simulink model "ModeInt"  (R2018b)
settings: Solver=FixedStepDiscrete  StartTime=0.0  StopTime=10.0  FixedStep=0.01  RelTol=1e-3
undefined symbols (not defined in the file or in its folder): c, CmprtMdHMIReqTp1, e, IfVeSMSeStNumConfig, MdReqTp1
(part 2 of 4)

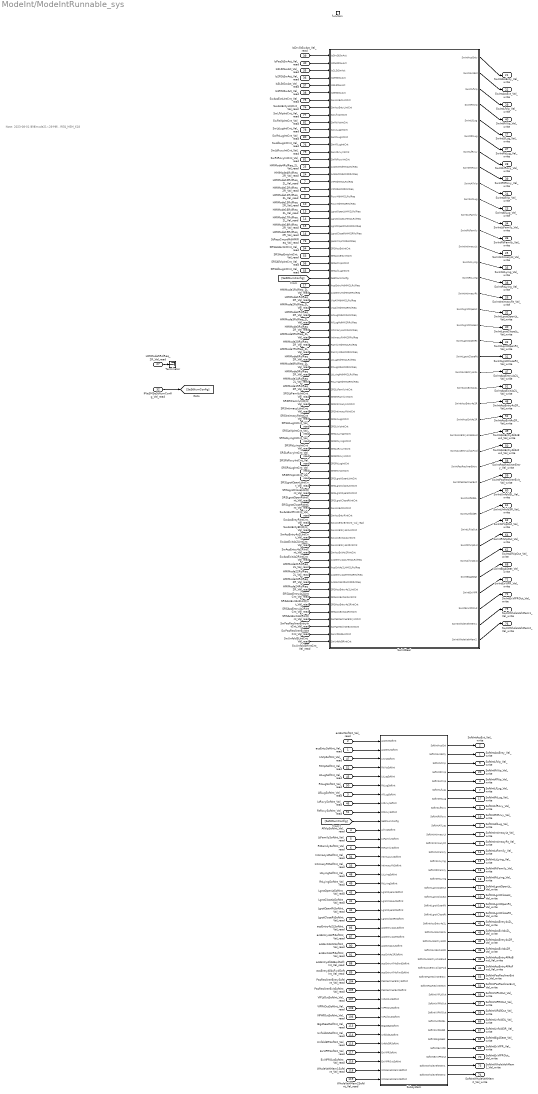
== system ModeInt/ModeIntRunnable_sys ==
  note: Note:
      | 2023-08-01:新增mode21~26中断，REQ_MSM_618
  acsEntySoftInt_Val_read : Inport
  acsExtSoftInt_Val_read : Inport  Port=2
  AllLugSoftInt_Val_read : Inport  Port=3
  AllVipSoftInt_Val_read : Inport  Port=4
  LtFamilySoftInt_Val_read : Inport  Port=5
  RtFamilySoftInt_Val_read : Inport  Port=6
  HMIMode10RclReq_2L_Val_read : Inport  Port=7
  HMIMode11RclReq_2L_Val_read : Inport  Port=8
  HMIMode12RclReq_2R_Val_read : Inport  Port=9
  HMIMode13RclReq_2R_Val_read : Inport  Port=10
  HMIMode14RclReq_2L_Val_read : Inport  Port=11
  HMIMode15RclReq_2R_Val_read : Inport  Port=12
  HMIMode16RclReq_2L_Val_read : Inport  Port=13
  HMIMode17RclReq_2L_Val_read : Inport  Port=14
  HMIMode18RclReq_2R_Val_read : Inport  Port=15
  HMIMode19RclReq_2R_Val_read : Inport  Port=16
  HMIMode1RclReq_2L_Val_read : Inport  Port=17
  HMIMode1RclReq_2R_Val_read : Inport  Port=18
  HMIMode20RclReq_2R_Val_read : Inport  Port=19
  HMIMode2RclReq_2L_Val_read : Inport  Port=20
  HMIMode2RclReq_2R_Val_read : Inport  Port=21
  HMIMode3RclReq_2L_Val_read : Inport  Port=22
  HMIMode3RclReq_2R_Val_read : Inport  Port=23
  HMIMode4RclReq_2R_Val_read : Inport  Port=24
  HMIMode4RclReq_2L_Val_read : Inport  Port=25
  HMIMode5RclReq_2L_Val_read : Inport  Port=26
  HMIMode5RclReq_2R_Val_read : Inport  Port=27
  HMIMode6RclReq_2R_Val_read : Inport  Port=28
  HMIMode7RclReq_2L_Val_read : Inport  Port=29
  HMIMode8RclReq_2L_Val_read : Inport  Port=30
  HMIMode9RclReq_2R_Val_read : Inport  Port=31
  IfVeSMSeStNumConfig_Val_read : Inport  Port=32
  IntimacyRtSoftInt_Val_read : Inport  Port=33
  IntimacyLtSoftInt_Val_read : Inport  Port=34
  Is2LStSwAct_Val_read : Inport  Port=35
  Is2RStSwAct_Val_read : Inport  Port=36
  Is3LStSwAct_Val_read : Inport  Port=37
  Is3RStSwAct_Val_read : Inport  Port=38
  IsDrvStSwAct_Val_read : Inport  Port=39
  IsPasStSwAct_Val_read : Inport  Port=40
  LgrstCloseLtSoftInt_Val_read : Inport  Port=41
  LgrstCloseRtSoftInt_Val_read : Inport  Port=42
  LgrstOpenLtSoftInt_Val_read : Inport  Port=43
  LgrstOpenRtSoftInt_Val_read : Inport  Port=44
  LtLugSoftInt_Val_read : Inport  Port=45
  LtRcvySoftInt_Val_read : Inport  Port=46
  LtVipSoftInt_Val_read : Inport  Port=47
  LtLyingSoftInt_Val_read : Inport  Port=48
  RtLyingSoftInt_Val_read : Inport  Port=49
  RtLugSoftInt_Val_read : Inport  Port=50
  RtRcvySoftInt_Val_read : Inport  Port=51
  RtVipSoftInt_Val_read : Inport  Port=52
  SRSAcsEntyIntCnt_Val_read : Inport  Port=53
  SRSAcsExtIntCnt_Val_read : Inport  Port=54
  SRSAllLugIntCnt_Val_read : Inport  Port=55
  SRSAllVipIntCnt_Val_read : Inport  Port=56
  SRSLtFamilyIntCnt_Val_read : Inport  Port=57
  SRSRtFamilyIntCnt_Val_read : Inport  Port=58
  SRSIntimacyLtIntCnt_Val_read : Inport  Port=59
  SRSIntimacyRtIntCnt_Val_read : Inport  Port=60
  SRSLtLugIntCnt_Val_read : Inport  Port=61
  SRSLtVipIntCnt_Val_read : Inport  Port=62
  SRSLgrstCloseLtIntCnt_Val_read : Inport  Port=63
  SRSLgrstCloseRtIntCnt_Val_read : Inport  Port=64
  SRSLgrstOpenLtIntCnt_Val_read : Inport  Port=65
  SRSLgrstOpenRtIntCnt_Val_read : Inport  Port=66
  SRSLtLyingIntCnt_Val_read : Inport  Port=67
  SRSRtLyingIntCnt_Val_read : Inport  Port=68
  SRSLtRcvyIntCnt_Val_read : Inport  Port=69
  SRSRtRcvyIntCnt_Val_read : Inport  Port=70
  SRSRtLugIntCnt_Val_read : Inport  Port=71
  SRSRtVipIntCnt_Val_read : Inport  Port=72
  StPassCmprtMdHMIReq_Val_read : Inport  Port=73
  SwAcsEntyLIntCnt_Val_read : Inport  Port=74
  SwAcsExtLIntCnt_Val_read : Inport  Port=75
  SwAllLugIntCnt_Val_read : Inport  Port=76
  SwLfVipIntCnt_Val_read : Inport  Port=77
  SwLtLugIntCnt_Val_read : Inport  Port=78
  SwLtRcvyIntCnt_Val_read : Inport  Port=79
  SwRtLugIntCnt_Val_read : Inport  Port=80
  SwRtRcvyIntCnt_Val_read : Inport  Port=81
  SwRtVipIntCnt_Val_read : Inport  Port=82
  SwAcsEntyRIntCnt_Val_read : Inport  Port=83
  SwAcsExtRIntCnt_Val_read : Inport  Port=84
  SwAcsEntyBIntCnt_Val_read : Inport  Port=85
  acsEntry4s2LSoftInt_Val_read : Inport  Port=86
  acsEntry4s2RSoftInt_Val_read : Inport  Port=87
  acsEntryAll4sBwdSoftInt_Val_read : Inport  Port=88
  acsEntryAll4sFwdSoftInt_Val_read : Inport  Port=89
  acsExit4s2LSoftInt_Val_read : Inport  Port=90
  acsExit4s2RSoftInt_Val_read : Inport  Port=91
  HMIMode21RclReq_2L_Val_read : Inport  Port=92
  HMIMode22RclReq_2L_Val_read : Inport  Port=93
  HMIMode23RclReq_2R_Val_read : Inport  Port=94
  HMIMode24RclReq_2R_Val_read : Inport  Port=95
  SRSAcsEntry4s2LIntCnt_Val_read : Inport  Port=96
  SRSAcsEntry4s2RIntCnt_Val_read : Inport  Port=97
  SRSAcsExit4s2LIntCnt_Val_read : Inport  Port=98
  SRSAcsExit4s2RIntCnt_Val_read : Inport  Port=99
  SwAcsEntry4s2LIntCnt_Val_read : Inport  Port=100
  SwAcsEntry4s2RIntCnt_Val_read : Inport  Port=101
  SwAcsExit4s2LIntCnt_Val_read : Inport  Port=102
  SwAcsExit4s2RIntCnt_Val_read : Inport  Port=103
  PasReclinerEntrySoftInt_Val_read : Inport  Port=104
  PasReclinerExitSoftInt_Val_read : Inport  Port=105
  VIPAllOutSoftInt_Val_read : Inport  Port=106
  VIPLtOutSoftInt_Val_read : Inport  Port=107
  VIPRtOutSoftInt_Val_read : Inport  Port=108
  SwPasReclinerEntryIntCnt_Val_read : Inport  Port=109
  SwPasReclinerExitIntCnt_Val_read : Inport  Port=110
  SwUnfold3LIntCnt_Val_read : Inport  Port=111
  SwUnfold3RIntCnt_Val_read : Inport  Port=112
  Big4SeatSoftInt_Val_read : Inport  Port=113
  Unfold3LSoftInt_Val_read : Inport  Port=114
  Unfold3RSoftInt_Val_read : Inport  Port=115
  ExVIPROutSoftInt_Val_read : Inport  Port=116
  ExVIPRSoftInt_Val_read : Inport  Port=117
  WholeVehMem1SoftInt_Val_read : Inport  Port=118
  WholeVehMem2SoftInt_Val_read : Inport  Port=119
  function : TriggerPort  TriggerType=function-call  VariantControl=(inherit)  SampleTimeType=periodic  SampleTime=-1
  Subsystem : Subsystem
  SwIntDeal : Subsystem
  Terminator : Terminator
  SoftIntAcsEnty_Val_write : Outport
  SoftIntAcsExt_Val_write : Outport  Port=2
  SoftIntAllLug_Val_write : Outport  Port=3
  SoftIntAllVip_Val_write : Outport  Port=4
  SoftIntIntimacyLt_Val_write : Outport  Port=5
  SoftIntIntimacyRt_Val_write : Outport  Port=6
  SoftIntLfLug_Val_write : Outport  Port=7
  SoftIntLfRcvy_Val_write : Outport  Port=8
  SoftIntLfVip_Val_write : Outport  Port=9
  SoftIntLgrstCloseLt_Val_write : Outport  Port=10
  SoftIntLgrstCloseRt_Val_write : Outport  Port=11
  SoftIntLgrstOpenLt_Val_write : Outport  Port=12
  SoftIntLgrstOpenRt_Val_write : Outport  Port=13
  SoftIntLtFamily_Val_write : Outport  Port=14
  SoftIntLtLying_Val_write : Outport  Port=15
  SoftIntRtFamily_Val_write : Outport  Port=16
  SoftIntRtLug_Val_write : Outport  Port=17
  SoftIntRtLying_Val_write : Outport  Port=18
  SoftIntRtRcvy_Val_write : Outport  Port=19
  SoftIntRtVip_Val_write : Outport  Port=20
  SwIntAcsEnty_Val_write : Outport  Port=21
  SwIntAcsExt_Val_write : Outport  Port=22
  SwIntAllLug_Val_write : Outport  Port=23
  SwIntAllVip_Val_write : Outport  Port=24
  SwIntIntimacyLt_Val_write : Outport  Port=25
  SwIntIntimacyRt_Val_write : Outport  Port=26
  SwIntLfLug_Val_write : Outport  Port=27
  SwIntLfRcvy_Val_write : Outport  Port=28
  SwIntLfVip_Val_write : Outport  Port=29
  SwIntLgrstCloseLt_Val_write : Outport  Port=30
  SwIntLgrstCloseRt_Val_write : Outport  Port=31
  SwIntLgrstOpenLt_Val_write : Outport  Port=32
  SwIntLgrstOpenRt_Val_write : Outport  Port=33
  SwIntLtFamily_Val_write : Outport  Port=34
  SwIntLtLying_Val_write : Outport  Port=35
  SwIntRtFamily_Val_write : Outport  Port=36
  SwIntRtLug_Val_write : Outport  Port=37
  SwIntRtLying_Val_write : Outport  Port=38
  SwIntRtRcvy_Val_write : Outport  Port=39
  SwIntRtVip_Val_write : Outport  Port=40
  SoftIntAcsEntry4s2L_Val_write : Outport  Port=41
  SoftIntAcsEntry4s2R_Val_write : Outport  Port=42
  SoftIntAcsEntryAll4sBwd_Val_write : Outport  Port=43
  SoftIntAcsEntryAll4sFwd_Val_write : Outport  Port=44
  SoftIntAcsExit4s2L_Val_write : Outport  Port=45
  SoftIntAcsExit4s2R_Val_write : Outport  Port=46
  SwIntAcsEntry4s2L_Val_write : Outport  Port=47
  SwIntAcsEntry4s2R_Val_write : Outport  Port=48
  SwIntAcsEntryAll4sBwd_Val_write : Outport  Port=49
  SwIntAcsEntryAll4sFwd_Val_write : Outport  Port=50
  SwIntAcsExit4s2L_Val_write : Outport  Port=51
  SwIntAcsExit4s2R_Val_write : Outport  Port=52
  SoftIntPasReclinerEntry_Val_write : Outport  Port=53
  SoftIntPasReclinerExit_Val_write : Outport  Port=54
  SoftIntVIPAllOut_Val_write : Outport  Port=55
  SoftIntVIPLtOut_Val_write : Outport  Port=56
  SoftIntVIPRtOut_Val_write : Outport  Port=57
  SwIntPasReclinerEntry_Val_write : Outport  Port=58
  SwIntPasReclinerExit_Val_write : Outport  Port=59
  SwIntUnfold3L_Val_write : Outport  Port=60
  SwIntUnfold3R_Val_write : Outport  Port=61
  SwIntAllVipOut_Val_write : Outport  Port=62
  SwIntLfVipOut_Val_write : Outport  Port=63
  SwIntRtVipOut_Val_write : Outport  Port=64
  SoftIntBig4Seat_Val_write : Outport  Port=65
  SoftIntUnfold3L_Val_write : Outport  Port=66
  SoftIntUnfold3R_Val_write : Outport  Port=67
  SwIntBig4Seat_Val_write : Outport  Port=68
  SoftIntExVIPR_Val_write : Outport  Port=69
  SoftIntExVIPROut_Val_write : Outport  Port=70
  SwIntExVIPR_Val_write : Outport  Port=71
  SwIntExVIPROut_Val_write : Outport  Port=72
  SoftIntWholeVehMem1_Val_write : Outport  Port=73
  SoftIntWholeVehMem2_Val_write : Outport  Port=74
  SwIntWholeVehMem1_Val_write : Outport  Port=75
  SwIntWholeVehMem2_Val_write : Outport  Port=76
  wires:
  SwIntDeal/1(SwIntAcsEnty) -> SwIntAcsEnty_Val_write/1
  SwIntDeal/2(SwIntAcsExt) -> SwIntAcsExt_Val_write/1
  SwIntDeal/3(SwIntLfVip) -> SwIntLfVip_Val_write/1
  SwIntDeal/4(SwIntRtVip) -> SwIntRtVip_Val_write/1
  SwIntDeal/5(SwIntLfLug) -> SwIntLfLug_Val_write/1
  SwIntDeal/6(SwIntRtLug) -> SwIntRtLug_Val_write/1
  SwIntDeal/7(SwIntLfRcvy) -> SwIntLfRcvy_Val_write/1
  SwIntDeal/8(SwIntRtRcvy) -> SwIntRtRcvy_Val_write/1
  SwIntDeal/9(SwIntAllVip) -> SwIntAllVip_Val_write/1
  SwIntDeal/10(SwIntAllLug) -> SwIntAllLug_Val_write/1
  SwIntDeal/11(SwIntLtFamily) -> SwIntLtFamily_Val_write/1
  SwIntDeal/12(SwIntRtFamily) -> SwIntRtFamily_Val_write/1
  SwIntDeal/13(SwIntIntimacyLt) -> SwIntIntimacyLt_Val_write/1
  SwIntDeal/14(SwIntLtLying) -> SwIntLtLying_Val_write/1
  SwIntDeal/15(SwIntRtLying) -> SwIntRtLying_Val_write/1
  SwIntDeal/16(SwIntIntimacyRt) -> SwIntIntimacyRt_Val_write/1
  SwIntDeal/17(SwIntLgrstOpenLt) -> SwIntLgrstOpenLt_Val_write/1
  SwIntDeal/18(SwIntLgrstCloseLt) -> SwIntLgrstCloseLt_Val_write/1
  SwIntDeal/19(SwIntLgrstOpenRt) -> SwIntLgrstOpenRt_Val_write/1
  SwIntDeal/20(SwIntLgrstCloseRt) -> SwIntLgrstCloseRt_Val_write/1
  IsDrvStSwAct_Val_read/1 -> SwIntDeal/1(IsDrvStSwAct)
  IsPasStSwAct_Val_read/1 -> SwIntDeal/2(IsPasStSwAct)
  Is2LStSwAct_Val_read/1 -> SwIntDeal/3(Is2LStSwAct)
  Is2RStSwAct_Val_read/1 -> SwIntDeal/4("Is2RStSwAct ")
  Is3LStSwAct_Val_read/1 -> SwIntDeal/5("Is3LStSwAct ")
  Is3RStSwAct_Val_read/1 -> SwIntDeal/6("Is3RStSwAct ")
  StPassCmprtMdHMIReq_Val_read/1 -> SwIntDeal/26(passCmprtMdHMIReq)
  SwAcsEntyLIntCnt_Val_read/1 -> SwIntDeal/8("SwAcsEntyLIntCnt ")
  SwAcsExtLIntCnt_Val_read/1 -> SwIntDeal/7(SwAcsExtLIntCnt)
  SwLfVipIntCnt_Val_read/1 -> SwIntDeal/9("SwLfVipIntCnt ")
  SwRtVipIntCnt_Val_read/1 -> SwIntDeal/10(SwRtVipIntCnt)
  SwLtLugIntCnt_Val_read/1 -> SwIntDeal/11(SwLtLugIntCnt)
  SwRtLugIntCnt_Val_read/1 -> SwIntDeal/12(SwRtLugIntCnt)
  SwAllLugIntCnt_Val_read/1 -> SwIntDeal/13(SwAllLugIntCnt)
  SwLtRcvyIntCnt_Val_read/1 -> SwIntDeal/14(SwLtRcvyIntCnt)
  SwRtRcvyIntCnt_Val_read/1 -> SwIntDeal/15(SwRtRcvyIntCnt)
  SRSLtFamilyIntCnt_Val_read/1 -> SwIntDeal/46(SRSLtFamilyIntCnt)
  SRSRtFamilyIntCnt_Val_read/1 -> SwIntDeal/47(SRSRtFamilyIntCnt)
  SRSIntimacyLtIntCnt_Val_read/1 -> SwIntDeal/48(SRSIntimacyLtIntCnt)
  SRSIntimacyRtIntCnt_Val_read/1 -> SwIntDeal/49(SRSIntimacyRtIntCnt)
  SRSLtLugIntCnt_Val_read/1 -> SwIntDeal/50(SRSLtLugIntCnt)
  SRSLtVipIntCnt_Val_read/1 -> SwIntDeal/51(SRSLtVipIntCnt)
  SRSLtLyingIntCnt_Val_read/1 -> SwIntDeal/52(SRSLtLyingIntCnt)
  SRSRtLyingIntCnt_Val_read/1 -> SwIntDeal/53(SRSRtLyingIntCnt)
  SRSLtRcvyIntCnt_Val_read/1 -> SwIntDeal/54(SRSLtRcvyIntCnt)
  SRSRtRcvyIntCnt_Val_read/1 -> SwIntDeal/55(SRSRtRcvyIntCnt)
  SRSRtLugIntCnt_Val_read/1 -> SwIntDeal/56(SRSRtLugIntCnt)
  SRSRtVipIntCnt_Val_read/1 -> SwIntDeal/57(SRSRtVipIntCnt)
  SRSLgrstCloseLtIntCnt_Val_read/1 -> SwIntDeal/59(SRSLgrstCloseLtIntCnt)
  SRSLgrstCloseRtIntCnt_Val_read/1 -> SwIntDeal/61(SRSLgrstCloseRtIntCnt)
  SRSLgrstOpenLtIntCnt_Val_read/1 -> SwIntDeal/58(SRSLgrstOpenLtIntCnt)
  SRSLgrstOpenRtIntCnt_Val_read/1 -> SwIntDeal/60(SRSLgrstOpenRtIntCnt)
  SRSAcsExtIntCnt_Val_read/1 -> SwIntDeal/27(SRSAcsExtIntCnt)
  SRSAcsEntyIntCnt_Val_read/1 -> SwIntDeal/28(SRSAcsEntyIntCnt)
  SRSAllLugIntCnt_Val_read/1 -> SwIntDeal/30(SRSAllLugIntCnt)
  SRSAllVipIntCnt_Val_read/1 -> SwIntDeal/29(SRSAllVipIntCnt)
  HMIMode1RclReq_2L_Val_read/1 -> SwIntDeal/32(AcsEntryMdHMI2LRclReq)
  HMIMode1RclReq_2R_Val_read/1 -> SwIntDeal/33(AcsEntryMdHMI2RRclReq)
  HMIMode4RclReq_2L_Val_read/1 -> SwIntDeal/16(AcsExtMdHMI2LRclReq)
  HMIMode4RclReq_2R_Val_read/1 -> SwIntDeal/17(AcsExtMdHMI2RRclReq)
  HMIMode10RclReq_2L_Val_read/1 -> SwIntDeal/18(VIPMdHMI2LRclReq)
  HMIMode12RclReq_2R_Val_read/1 -> SwIntDeal/19(VIPMdHMI2RRclReq)
  HMIMode11RclReq_2L_Val_read/1 -> SwIntDeal/20(RcvyMdHMI2LRclReq)
  HMIMode13RclReq_2R_Val_read/1 -> SwIntDeal/21(RcvyMdHMI2RRclReq)
  HMIMode2RclReq_2L_Val_read/1 -> SwIntDeal/34(VipAllMdHMI2LRclReq)
  HMIMode2RclReq_2R_Val_read/1 -> SwIntDeal/35(VipAllMdHMI2RRclReq)
  HMIMode3RclReq_2L_Val_read/1 -> SwIntDeal/36(AllLugMdHMI2LRclReq)
  HMIMode3RclReq_2R_Val_read/1 -> SwIntDeal/37(AllLugMdHMI2RRclReq)
  HMIMode5RclReq_2L_Val_read/1 -> SwIntDeal/38(IntimacyLHMI2LRclReq)
  HMIMode20RclReq_2R_Val_read/1 -> SwIntDeal/39(IntimacyRHMI2RRclReq)
  HMIMode7RclReq_2L_Val_read/1 -> SwIntDeal/40(FamilyMdHMI2LRclReq)
  HMIMode6RclReq_2R_Val_read/1 -> SwIntDeal/41(FamilyMdHMI2RRclReq)
  HMIMode8RclReq_2L_Val_read/1 -> SwIntDeal/42(LtLugMdHMI2LRclReq)
  HMIMode9RclReq_2R_Val_read/1 -> SwIntDeal/43(RtLugMdHMI2RRclReq)
  HMIMode14RclReq_2L_Val_read/1 -> SwIntDeal/44(LtLyingMdHMI2LRclReq)
  HMIMode15RclReq_2R_Val_read/1 -> SwIntDeal/45(RtLyingMdHMI2RRclReq)
  HMIMode16RclReq_2L_Val_read/1 -> SwIntDeal/22(LgrstOpenLtHMI2LRclReq)
  HMIMode17RclReq_2L_Val_read/1 -> SwIntDeal/23(LgrstCloseLtHMI2LRclReq)
  HMIMode18RclReq_2R_Val_read/1 -> SwIntDeal/24(LgrstOpenRtHMI2RRclReq)
  HMIMode19RclReq_2R_Val_read/1 -> SwIntDeal/25(LgrstCloseRtHMI2RRclReq)
  HMIMode5RclReq_2R_Val_read/1 -> Terminator/1
  Subsystem/2(SoftIntAcsEnty) -> SoftIntAcsEnty_Val_write/1
  Subsystem/1(SoftIntAcsExt) -> SoftIntAcsExt_Val_write/1
  Subsystem/10(SoftIntAllLug) -> SoftIntAllLug_Val_write/1
  Subsystem/5(SoftIntAllVip) -> SoftIntAllVip_Val_write/1
  Subsystem/3(SoftIntLfVip) -> SoftIntLfVip_Val_write/1
  Subsystem/4(SoftIntRtVip) -> SoftIntRtVip_Val_write/1
  IfVeSMSeStNumConfig_Val_read/1 -> [SeStNumConfig]
  [SeStNumConfig] -> SwIntDeal/31(SeStNumConfig)
  [SeStNumConfig] -> Subsystem/10(SeStNumConfig)
  acsExtSoftInt_Val_read/1 -> Subsystem/1(acsExtSoftInt)
  acsEntySoftInt_Val_read/1 -> Subsystem/2(acsEntySoftInt)
  AllLugSoftInt_Val_read/1 -> Subsystem/7(AllLugSoftInt)
  AllVipSoftInt_Val_read/1 -> Subsystem/11(AllVipSoftInt)
  LtFamilySoftInt_Val_read/1 -> Subsystem/12(LtFamilySoftInt)
  RtFamilySoftInt_Val_read/1 -> Subsystem/13(RtFamilySoftInt)
  LtRcvySoftInt_Val_read/1 -> Subsystem/8(LtRcvySoftInt)
  RtRcvySoftInt_Val_read/1 -> Subsystem/9(RtRcvySoftInt)
  RtLugSoftInt_Val_read/1 -> Subsystem/6(RtLugSoftInt)
  LtLugSoftInt_Val_read/1 -> Subsystem/5(LtLugSoftInt)
  RtVipSoftInt_Val_read/1 -> Subsystem/4(RtVipSoftInt)
  LtVipSoftInt_Val_read/1 -> Subsystem/3(LtVipSoftInt)
  LtLyingSoftInt_Val_read/1 -> Subsystem/16(LtLyingSoftInt)
  RtLyingSoftInt_Val_read/1 -> Subsystem/17(RtLyingSoftInt)
  IntimacyLtSoftInt_Val_read/1 -> Subsystem/14(IntimacyLtSoftInt)
  IntimacyRtSoftInt_Val_read/1 -> Subsystem/15(IntimacyRtSoftInt)
  LgrstCloseLtSoftInt_Val_read/1 -> Subsystem/19(LgrstCloseLtSoftInt)
  LgrstOpenLtSoftInt_Val_read/1 -> Subsystem/18(LgrstOpenLtSoftInt)
  LgrstOpenRtSoftInt_Val_read/1 -> Subsystem/20(LgrstOpenRtSoftInt)
  LgrstCloseRtSoftInt_Val_read/1 -> Subsystem/21(LgrstCloseRtSoftInt)
  Subsystem/6(SoftIntLfLug) -> SoftIntLfLug_Val_write/1
  Subsystem/7(SoftIntRtLug) -> SoftIntRtLug_Val_write/1
  Subsystem/8(SoftIntLfRcvy) -> SoftIntLfRcvy_Val_write/1
  Subsystem/9(SoftIntRtRcvy) -> SoftIntRtRcvy_Val_write/1
  Subsystem/16(SoftIntRtLying) -> SoftIntRtLying_Val_write/1
  Subsystem/11(SoftIntIntimacyLt) -> SoftIntIntimacyLt_Val_write/1
  Subsystem/12(SoftIntIntimacyRt) -> SoftIntIntimacyRt_Val_write/1
  Subsystem/13(SoftIntLtFamily) -> SoftIntLtFamily_Val_write/1
  Subsystem/14(SoftIntLtLying) -> SoftIntLtLying_Val_write/1
  Subsystem/15(SoftIntRtFamily) -> SoftIntRtFamily_Val_write/1
  Subsystem/17(SoftIntLgrstOpenLt) -> SoftIntLgrstOpenLt_Val_write/1
  Subsystem/18(SoftIntLgrstCloseLt) -> SoftIntLgrstCloseLt_Val_write/1
  Subsystem/19(SoftIntLgrstOpenRt) -> SoftIntLgrstOpenRt_Val_write/1
  Subsystem/20(SoftIntLgrstCloseRt) -> SoftIntLgrstCloseRt_Val_write/1
  SwAcsExtRIntCnt_Val_read/1 -> SwIntDeal/62(SwAcsExtRIntCnt)
  SwAcsEntyRIntCnt_Val_read/1 -> SwIntDeal/63(SwAcsEntyRIntCnt)
  SwAcsEntyBIntCnt_Val_read/1 -> SwIntDeal/64(SwAcsEntyBIntCnt_Val_read)
  SwAcsEntry4s2LIntCnt_Val_read/1 -> SwIntDeal/65(SwAcsEntry4s2LIntCnt)
  SwAcsExit4s2LIntCnt_Val_read/1 -> SwIntDeal/66(SwAcsExit4s2LIntCnt)
  SwAcsEntry4s2RIntCnt_Val_read/1 -> SwIntDeal/67(SwAcsEntry4s2RIntCnt)
  SwAcsExit4s2RIntCnt_Val_read/1 -> SwIntDeal/68(SwAcsExit4s2RIntCnt)
  HMIMode21RclReq_2L_Val_read/1 -> SwIntDeal/69(AcsEntry4s2LHMI2LRclReq)
  HMIMode22RclReq_2L_Val_read/1 -> SwIntDeal/70(AcsExit4s2LHMI2LRclReq)
  HMIMode23RclReq_2R_Val_read/1 -> SwIntDeal/71(AcsEntry4s2RHMI2RRclReq)
  HMIMode24RclReq_2R_Val_read/1 -> SwIntDeal/72(AcsExit4s2RHMI2RRclReq)
  SRSAcsEntry4s2LIntCnt_Val_read/1 -> SwIntDeal/73(SRSAcsEntry4s2LIntCnt)
  SRSAcsExit4s2LIntCnt_Val_read/1 -> SwIntDeal/74(SRSAcsExit4s2LIntCnt)
  SRSAcsEntry4s2RIntCnt_Val_read/1 -> SwIntDeal/75(SRSAcsEntry4s2RIntCnt)
  SRSAcsExit4s2RIntCnt_Val_read/1 -> SwIntDeal/76(SRSAcsExit4s2RIntCnt)
  SwIntDeal/21(SwIntAcsEntry4s2L) -> SwIntAcsEntry4s2L_Val_write/1
  SwIntDeal/22(SwIntAcsExit4s2L) -> SwIntAcsExit4s2L_Val_write/1
  SwIntDeal/23(SwIntAcsEntry4s2R) -> SwIntAcsEntry4s2R_Val_write/1
  SwIntDeal/24(SwIntAcsExit4s2R) -> SwIntAcsExit4s2R_Val_write/1
  SwIntDeal/25(SwIntAcsEntryAll4sBwd) -> SwIntAcsEntryAll4sBwd_Val_write/1
  SwIntDeal/26(SwIntAcsEntryAll4sFwd) -> SwIntAcsEntryAll4sFwd_Val_write/1
  Subsystem/21(SoftIntAcsEntry4s2L) -> SoftIntAcsEntry4s2L_Val_write/1
  Subsystem/22(SoftIntAcsExit4s2L) -> SoftIntAcsExit4s2L_Val_write/1
  Subsystem/23(SoftIntAcsEntry4s2R) -> SoftIntAcsEntry4s2R_Val_write/1
  Subsystem/24(SoftIntAcsExit4s2R) -> SoftIntAcsExit4s2R_Val_write/1
  Subsystem/25(SoftIntAcsEntryAll4sBwd) -> SoftIntAcsEntryAll4sBwd_Val_write/1
  Subsystem/26(SoftIntAcsEntryAll4sFwd) -> SoftIntAcsEntryAll4sFwd_Val_write/1
  acsEntry4s2LSoftInt_Val_read/1 -> Subsystem/22(acsEntry4s2LSoftInt)
  acsEntry4s2RSoftInt_Val_read/1 -> Subsystem/23(" acsEntry4s2RSoftInt")
  acsEntryAll4sBwdSoftInt_Val_read/1 -> Subsystem/26(acsEntryAll4sBwdSoftInt)
  acsEntryAll4sFwdSoftInt_Val_read/1 -> Subsystem/27(acsEntryAll4sFwdSoftInt)
  acsExit4s2LSoftInt_Val_read/1 -> Subsystem/24(acsExit4s2LSoftInt)
  acsExit4s2RSoftInt_Val_read/1 -> Subsystem/25(acsExit4s2RSoftInt)
  SwPasReclinerEntryIntCnt_Val_read/1 -> SwIntDeal/77(SwPasReclinerEntryIntCnt)
  SwPasReclinerExitIntCnt_Val_read/1 -> SwIntDeal/78(SwPasReclinerExitIntCnt)
  SwUnfold3LIntCnt_Val_read/1 -> SwIntDeal/79(SwUnfold3LIntCnt)
  SwUnfold3RIntCnt_Val_read/1 -> SwIntDeal/80(SwUnfold3RIntCnt)
  PasReclinerEntrySoftInt_Val_read/1 -> Subsystem/28(PasReclinerEntrySoftInt)
  PasReclinerExitSoftInt_Val_read/1 -> Subsystem/29(PasReclinerExitSoftInt)
  VIPLtOutSoftInt_Val_read/1 -> Subsystem/30(VIPLtOutSoftInt)
  VIPRtOutSoftInt_Val_read/1 -> Subsystem/31(VIPRtOutSoftInt)
  VIPAllOutSoftInt_Val_read/1 -> Subsystem/32(VIPAllOutSoftInt)
  Subsystem/27(SoftIntPasReclinerEntry) -> SoftIntPasReclinerEntry_Val_write/1
  Subsystem/28(SoftIntPasReclinerExit) -> SoftIntPasReclinerExit_Val_write/1
  Subsystem/31(SoftIntVIPAllOut) -> SoftIntVIPAllOut_Val_write/1
  Subsystem/29(SoftIntVIPLtOut) -> SoftIntVIPLtOut_Val_write/1
  Subsystem/30(SoftIntVIPRtOut) -> SoftIntVIPRtOut_Val_write/1
  SwIntDeal/27(SwIntPasReclinerEntry) -> SwIntPasReclinerEntry_Val_write/1
  SwIntDeal/28(SwIntPasReclinerExit) -> SwIntPasReclinerExit_Val_write/1
  SwIntDeal/29(SwIntUnfold3L) -> SwIntUnfold3L_Val_write/1
  SwIntDeal/30(SwIntUnfold3R) -> SwIntUnfold3R_Val_write/1
  SwIntDeal/33(SwIntAllVipOut) -> SwIntAllVipOut_Val_write/1
  SwIntDeal/31(SwIntLfVipOut) -> SwIntLfVipOut_Val_write/1
  SwIntDeal/32(SwIntRtVipOut) -> SwIntRtVipOut_Val_write/1
  SwIntDeal/34(SwIntBig4Seat) -> SwIntBig4Seat_Val_write/1
  Big4SeatSoftInt_Val_read/1 -> Subsystem/33(Big4SeatSoftInt)
  Unfold3LSoftInt_Val_read/1 -> Subsystem/34(Unfold3LSoftInt)
  Unfold3RSoftInt_Val_read/1 -> Subsystem/35(Unfold3RSoftInt)
  Subsystem/32(SoftIntUnfold3L) -> SoftIntUnfold3L_Val_write/1
  Subsystem/33(SoftIntUnfold3R) -> SoftIntUnfold3R_Val_write/1
  Subsystem/34(SoftIntBig4Seat) -> SoftIntBig4Seat_Val_write/1
  SwIntDeal/35(SwIntExVIPR) -> SwIntExVIPR_Val_write/1
  SwIntDeal/36(SwIntExVIPROut) -> SwIntExVIPROut_Val_write/1
  ExVIPRSoftInt_Val_read/1 -> Subsystem/36(ExVIPRSoftInt)
  ExVIPROutSoftInt_Val_read/1 -> Subsystem/37(ExVIPROutSoftInt)
  Subsystem/35(SoftIntExVIPR) -> SoftIntExVIPR_Val_write/1
  Subsystem/36(SoftIntExVIPROut) -> SoftIntExVIPROut_Val_write/1
  SwIntDeal/37(SwIntWholeVehMem1) -> SwIntWholeVehMem1_Val_write/1
  SwIntDeal/38(SwIntWholeVehMem2) -> SwIntWholeVehMem2_Val_write/1
  WholeVehMem1SoftInt_Val_read/1 -> Subsystem/38(WholeVehMem1SoftInt)
  WholeVehMem2SoftInt_Val_read/1 -> Subsystem/39(WholeVehMem2SoftInt)
  Subsystem/38(SoftIntWholeVehMem2) -> SoftIntWholeVehMem2_Val_write/1
  Subsystem/37(SoftIntWholeVehMem1) -> SoftIntWholeVehMem1_Val_write/1

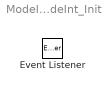
== system ModeInt/ModeInt_Init ==
  Event Listener : EventListener  EventName=reset
